simulink model "control_lab_5555"  (R2019b)
settings: Solver=FixedStepAuto  StartTime=0.0  StopTime=16  FixedStep=0.001  RelTol=1e-3
settings Model: Creator=Abdurrahman  LastModifiedBy=Abdurrahman

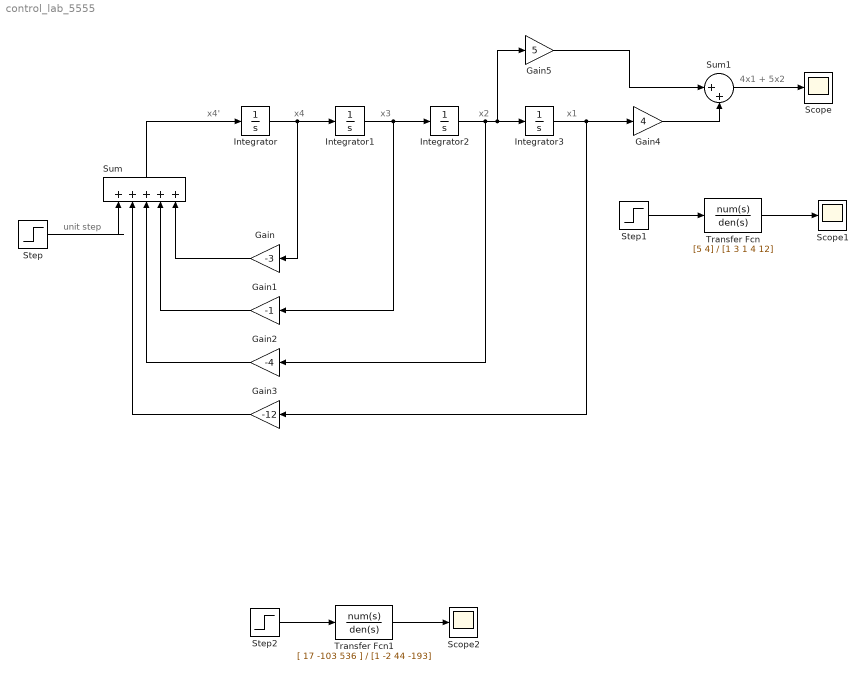
== system control_lab_5555 ==
  note: unit step
  note: 4x1 + 5x2
  note: x1
  note: x2
  note: x3
  note: x4
  note: x4'
  Gain : Gain  Gain=-3
  Gain1 : Gain  Gain=-1
  Gain2 : Gain  Gain=-4
  Gain3 : Gain  Gain=-12
  Gain4 : Gain  Gain=4
  Gain5 : Gain  Gain=5
  Integrator{,1..3} (4 alike) : Integrator
  Scope : Scope
  Scope1 : Scope
  Scope2 : Scope
  Step : Step  SampleTime=0
  Step1 : Step  SampleTime=0
  Step2 : Step  SampleTime=0
  Sum : Sum  Inputs=|+++++
  Sum1 : Sum  Inputs=|++
  Transfer Fcn : TransferFcn  Numerator=[5 4]  Denominator=[1 3 1 4 12]
  Transfer Fcn1 : TransferFcn  Numerator=[ 17 -103 536 ]  Denominator=[1 -2 44 -193]
  wires:
  Integrator/1 -> Integrator1/1, Gain/1
  Integrator1/1 -> Gain1/1, Integrator2/1
  Integrator2/1 -> Gain2/1, Gain5/1, Integrator3/1
  Integrator3/1 -> Gain4/1, Gain3/1
  Sum/1 -> Integrator/1
  Gain/1 -> Sum/5
  Gain1/1 -> Sum/4
  Gain2/1 -> Sum/3
  Gain3/1 -> Sum/2
  Step/1 -> Sum/1
  Gain5/1 -> Sum1/1
  Gain4/1 -> Sum1/2
  Sum1/1 -> Scope/1
  Step1/1 -> Transfer Fcn/1
  Transfer Fcn/1 -> Scope1/1
  Step2/1 -> Transfer Fcn1/1
  Transfer Fcn1/1 -> Scope2/1
